simulink model "Lab1simulink"  (R2024b)
settings: Solver=VariableStepAuto  StartTime=0.0  StopTime=8.0  RelTol=1e-3
undefined symbols (not defined in the file or in its folder): pulse
libraries: simulink x1
settings Model: Creator=Ahmed AlAlwani  LastModifiedBy=ANDALOS
settings DebuggingCC: UnconnectedInputMsg=warning  UnconnectedOutputMsg=warning  UnconnectedLineMsg=warning
settings ModelReferenceCC: EnableRefExpFcnMdlSchedulingChecks=on
settings RTWCC: GPUComputeCapability=3.5  DLArmComputeVersion=19.05

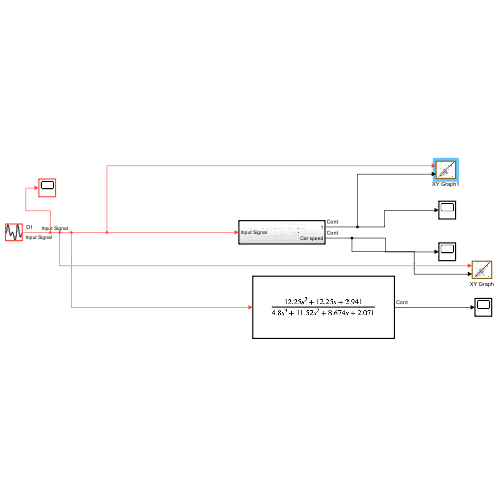
[thumbnail: Simulink's stored preview of the top-level diagram]
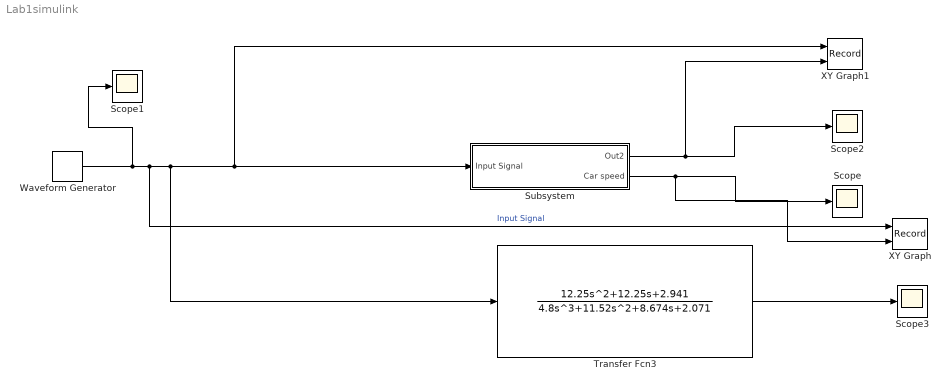
== system Lab1simulink ==
  Scope{,1..3} (4 alike) : Scope
  Subsystem : Subsystem
  Transfer Fcn3 : TransferFcn  Numerator=[0 12.25 12.25 2.941]  Denominator=[4.8 11.52 8.674 2.071]
  Waveform Generator : simulink/Sources/Waveform Generator  OutMin=[]  OutMax=[]  OutDataTypeStr=double  SelectedSignal=1  Signals=pulse(1,1,2)  BlockNames=MultiportSwitch_1bab38db7f814d7  SampleTime=0.1
  XY Graph : Record  FileSettingsInternal="{\"entries\":[{\"content\":{\"excelSettings\":{\"content\":{},\"type\":\"Streamout.ExcelSettings\"}},\"type\":\"Streamout.FileSettingStorage\",\"uuid\":\"\"}],\"packageUris\":[\"http:\\/\\/schema.mathworks.com\\/mf0\\/streamout_blocks\\/R2020a\"],\"version\":\"1.0\"}"  Layout=[1 1]  SignalsInternal="{\"entries\":[{\"content\":{\"signals\":[{\"content\":{\"blockPath\":[],\"dimensions\":[1],\"domain\":\"\",\"lineColor\":\"#a2142f\",\"plots\":[ 1 ],\"port\":1,\"sid\":[\"\"],\"signalID\":1,\"signalName\":\"Input Signal\"},\"type\":\"RecordBlkView.Signal\",\"uuid\":\"\"},{\"content\":{\"blockPath\":[],\"dimensions\":[1],\"domain\":\"\",\"lineColor\":\"#139fff\",\"plots\":[ 1 ],\"port\":2,\"sid\":[\"\"],\"signalID\":2,\"signalName\":\"Subsystem:2\"},\"type\":\"RecordBlkView.Signal\",\"uuid\":\"\"}]},\"type\":\"RecordBlkView.InputSignals\",\"uuid\":\"\"}],\"packageUris\":[\"http:\\/\\/schema.mathworks.com\\/mf0\\/streamout_blocks\\/R2020a\"],\"version\":\"1.0\"}"  VisualizationBindings="{\"xyplotplugin\":{\"info\":[{\"series\":[{\"bindingParametersList\":[{\"parameter\":\"X-Axis\",\"signalID\":1,\"signalName\":\"Input Signal\"},{\"parameter\":\"Y-Axis\",\"signalID\":2,\"signalName\":\"Subsystem:2\"}],\"seriesID\":0}],\"subplotID\":1}]}}"  CompatibilityTag=XY
  XY Graph1 : Record  FileSettingsInternal="{\"entries\":[{\"content\":{\"excelSettings\":{\"content\":{},\"type\":\"Streamout.ExcelSettings\"}},\"type\":\"Streamout.FileSettingStorage\",\"uuid\":\"\"}],\"packageUris\":[\"http:\\/\\/schema.mathworks.com\\/mf0\\/streamout_blocks\\/R2020a\"],\"version\":\"1.0\"}"  Layout=[1 1]  SignalsInternal="{\"entries\":[{\"content\":{\"signals\":[{\"content\":{\"blockPath\":[],\"dimensions\":[1],\"domain\":\"\",\"lineColor\":\"#a2142f\",\"plots\":[ 1 ],\"port\":1,\"sid\":[\"\"],\"signalID\":1,\"signalName\":\"Input Signal\"},\"type\":\"RecordBlkView.Signal\",\"uuid\":\"\"},{\"content\":{\"blockPath\":[],\"dimensions\":[1],\"domain\":\"\",\"lineColor\":\"#139fff\",\"plots\":[ 1 ],\"port\":2,\"sid\":[\"\"],\"signalID\":2,\"signalName\":\"Subsystem:1\"},\"type\":\"RecordBlkView.Signal\",\"uuid\":\"\"}]},\"type\":\"RecordBlkView.InputSignals\",\"uuid\":\"\"}],\"packageUris\":[\"http:\\/\\/schema.mathworks.com\\/mf0\\/streamout_blocks\\/R2020a\"],\"version\":\"1.0\"}"  VisualizationBindings="{\"xyplotplugin\":{\"info\":[{\"series\":[{\"bindingParametersList\":[{\"parameter\":\"X-Axis\",\"signalID\":1,\"signalName\":\"Input Signal\"},{\"parameter\":\"Y-Axis\",\"signalID\":2,\"signalName\":\"Subsystem:1\"}],\"seriesID\":0}],\"subplotID\":1}]}}"  CompatibilityTag=XY
  wires:
  Waveform Generator/1 -> Scope1/1, XY Graph/1, XY Graph1/1, Subsystem/1(Input Signal), Transfer Fcn3/1  "Input Signal"
  Transfer Fcn3/1 -> Scope3/1
  Subsystem/1(Out2) -> XY Graph1/2, Scope2/1
  Subsystem/2(Car speed) -> XY Graph/2, Scope/1

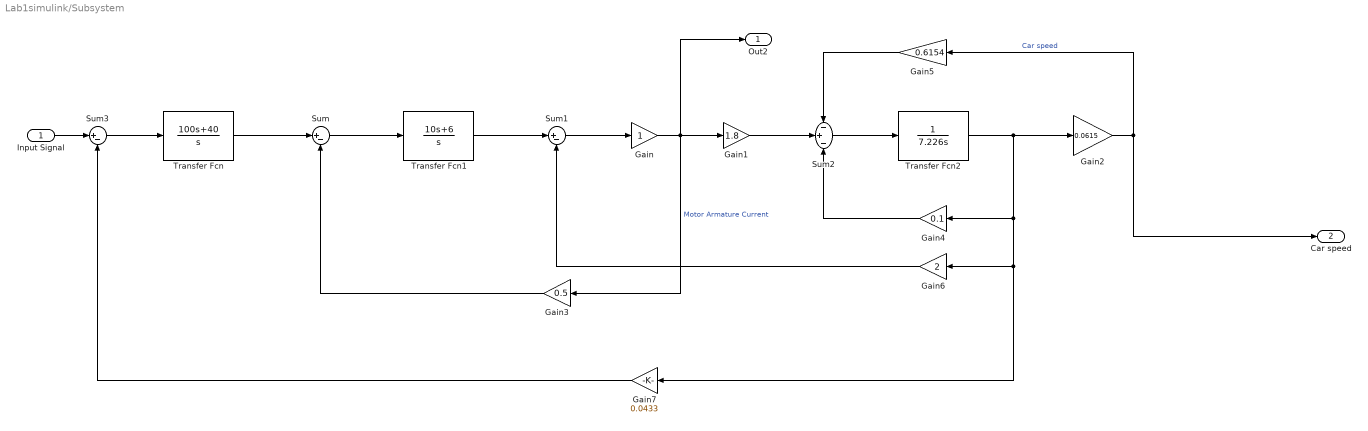
== system Lab1simulink/Subsystem ==
  Input Signal : Inport
  Gain : Gain
  Gain1 : Gain  Gain=1.8
  Gain2 : Gain  Gain=0.0615
  Gain3 : Gain  Gain=0.5
  Gain4 : Gain  Gain=0.1
  Gain5 : Gain  Gain=0.6154
  Gain6 : Gain  Gain=2
  Gain7 : Gain  Gain=0.0433
  Sum : Sum  Inputs=|+-
  Sum1 : Sum  Inputs=|+-
  Sum2 : Sum  Inputs=-+-
  Sum3 : Sum  Inputs=|+-
  Transfer Fcn : TransferFcn  Numerator=[100 40]  Denominator=[1 0]
  Transfer Fcn1 : TransferFcn  Numerator=[10 6]  Denominator=[1 0]
  Transfer Fcn2 : TransferFcn  Numerator=[0 1]  Denominator=[7.226 0]
  Out2 : Outport
  Car speed : Outport  Port=2
  wires:
  Gain1/1 -> Sum2/2
  Transfer Fcn1/1 -> Sum1/1
  Gain4/1 -> Sum2/3
  Sum2/1 -> Transfer Fcn2/1
  Gain5/1 -> Sum2/1
  Sum/1 -> Transfer Fcn1/1
  Gain2/1 -> Car speed/1, Gain5/1  "Car speed"
  Gain/1 -> Out2/1, Gain1/1, Gain3/1  "Motor Armature Current"
  Gain3/1 -> Sum/2
  Transfer Fcn2/1 -> Gain7/1, Gain6/1, Gain4/1, Gain2/1
  Sum3/1 -> Transfer Fcn/1
  Sum1/1 -> Gain/1
  Gain6/1 -> Sum1/2
  Transfer Fcn/1 -> Sum/1
  Gain7/1 -> Sum3/2
  Input Signal/1 -> Sum3/1
